simulink model "Air"  (R2026a)
settings: configuration reference "standardSILConfiguraitonParams" (kept outside this file)
undefined symbols (not defined in the file): F, gustDuration_sec, gustEnabled, gustStartTime_sec, Light, MIL, turbulenceEnabled, turbulenceEndTime_sec, turbulenceMinAirspeed_mps, turbulenceStartTime_sec, WIND_SOURCE, xWindInNED_mps, yWindInNED_mps, zWindInNED_mps
libraries: aerolibwind2 x3, simulink x2, aerolibatmos2 x1
settings Model: Creator=jerem  LastModifiedBy=Edison Altamirano
settings ConfigSetRef: SourceName=standardSILConfiguraitonParams  SourceLocation=Base Workspace

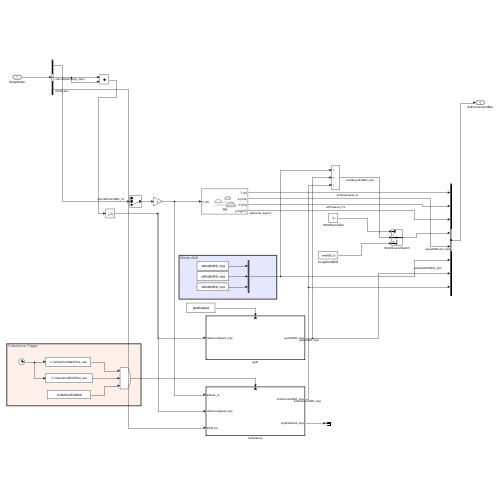
[thumbnail: Simulink's stored preview of the top-level diagram]
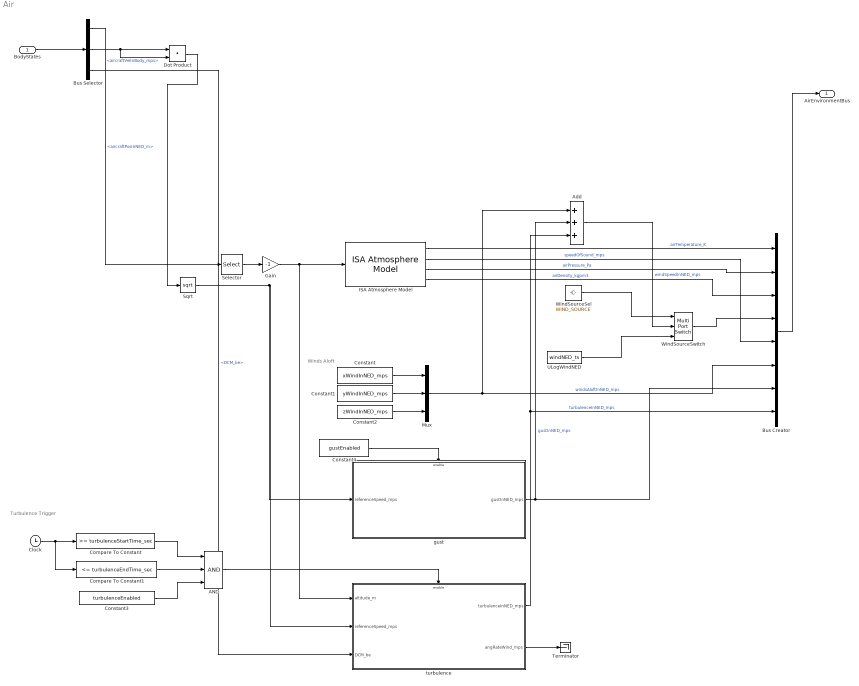
== system Air ==
  note: Turbulence Trigger
  note: Winds Aloft
  BodyStates : Inport  OutDataTypeStr=Bus: BodyStateBus
  AND : Logic  Inputs=3  IconShape=distinctive  AllPortsSameDT=off  OutDataTypeStr=boolean
  Add : Sum  Inputs=+++
  Bus Creator : BusCreator  Inputs=8  OutDataTypeStr=Bus: AirEnvironmentBus
  Bus Selector : BusSelector  OutputSignals=aircraftPosInNED_m,aircraftVelInBody_mps,DCM_be
  Clock : Clock
  Compare To Constant : simulink/Logic and Bit Operations/Compare To Constant  relop=>=  const=turbulenceStartTime_sec  OutDataTypeStr=boolean
  Compare To Constant1 : simulink/Logic and Bit Operations/Compare To Constant  relop=<=  const=turbulenceEndTime_sec  OutDataTypeStr=boolean
  Constant : Constant  Value=xWindInNED_mps
  Constant1 : Constant  Value=yWindInNED_mps
  Constant2 : Constant  Value=zWindInNED_mps
  Constant3 : Constant  Value=turbulenceEnabled
  Constant4 : Constant  Value=gustEnabled
  Dot Product : DotProduct  OutDataTypeStr=Inherit: Inherit via internal rule
  Gain : Gain  Gain=-1
  ISA Atmosphere Model : aerolibatmos2/ISA Atmosphere Model  useExtended=off  action=Warning  custom=off  viscosityOut=off  g=9.80665  gamma=1.4  R=287.0531  L=0.0065  h_trop=11000  h_strat=20000  rho0=1.225  P0=101325  T0=288.15  h0=0  S=110.4  Tref=273.15  muref=1.716e-5
  Mux : Mux  Inputs=3
  Selector : Selector  InputPortWidth=3  IndexOptions=Index vector (dialog)  Indices=3  OutputSizes=1
  Sqrt : Sqrt
  Terminator : Terminator
  ULogWindNED : FromWorkspace  VariableName=windNED_ts  OutputAfterFinalValue=Holding final value
  WindSourceSel : Constant  Value=WIND_SOURCE
  WindSourceSwitch : MultiPortSwitch  Inputs=2  SaturateOnIntegerOverflow=off  InputSameDT=off
  gust : Subsystem
  turbulence : Subsystem
  AirEnvironmentBus : Outport  OutDataTypeStr=Bus: AirEnvironmentBus
  wires:
  Constant1/1 -> Mux/2
  Constant/1 -> Mux/1
  Constant2/1 -> Mux/3
  Bus Creator/1 -> AirEnvironmentBus/1
  Selector/1 -> Gain/1
  ISA Atmosphere Model/3 -> Bus Creator/2  "airPressure_Pa"
  Bus Selector/1 -> Selector/1  "<aircraftPosInNED_m>"
  Gain/1 -> turbulence/1(altitude_m), ISA Atmosphere Model/1
  ISA Atmosphere Model/2 -> Bus Creator/5  "speedOfSound_mps"
  ISA Atmosphere Model/1 -> Bus Creator/1  "airTemperature_K"
  BodyStates/1 -> Bus Selector/1
  Mux/1 -> Bus Creator/6, Add/1  "windsAloftInNED_mps"
  ISA Atmosphere Model/4 -> Bus Creator/3  "airDensity_kgpm3"
  gust/1(gustInNED_mps) -> Bus Creator/7, Add/2  "gustInNED_mps"
  Add/1 -> WindSourceSwitch/2  "windSpeedInNED_mps"
  Bus Selector/2 -> Dot Product/2, Dot Product/1  "<aircraftVelInBody_mps>"
  Dot Product/1 -> Sqrt/1
  Bus Selector/3 -> turbulence/3(DCM_be)  "<DCM_be>"
  turbulence/1(turbulenceInNED_mps) -> Bus Creator/8, Add/3  "turbulenceInNED_mps"
  turbulence/2(angRateWind_mps) -> Terminator/1
  Sqrt/1 -> gust/1(referenceSpeed_mps), turbulence/2(referenceSpeed_mps)
  Clock/1 -> Compare To Constant1/1, Compare To Constant/1
  Compare To Constant/1 -> AND/1
  Compare To Constant1/1 -> AND/2
  AND/1 -> turbulence/Enable
  Constant3/1 -> AND/3
  Constant4/1 -> gust/Enable
  WindSourceSel/1 -> WindSourceSwitch/1
  ULogWindNED/1 -> WindSourceSwitch/3
  WindSourceSwitch/1 -> Bus Creator/4

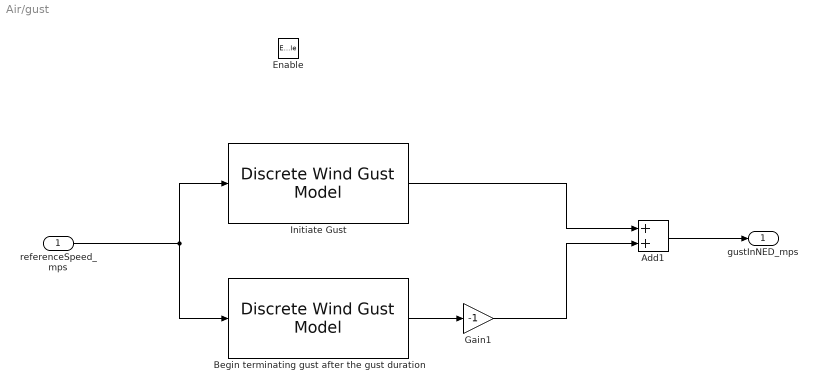
== system Air/gust ==
  referenceSpeed_mps : Inport
  Enable : EnablePort
  Add1 : Sum
  Begin terminating gust after the gust duration : aerolibwind2/Discrete Wind Gust Model  units=Metric (MKS)  Gx=on  Gy=on  Gz=on  t_0=gustStartTime_sec + gustDuration_sec  d_m=gustLength_m  v_m=gustAmplitude_mps
  Gain1 : Gain  Gain=-1
  Initiate Gust : aerolibwind2/Discrete Wind Gust Model  units=Metric (MKS)  Gx=on  Gy=on  Gz=on  t_0=gustStartTime_sec  d_m=gustLength_m  v_m=gustAmplitude_mps
  gustInNED_mps : Outport
  wires:
  referenceSpeed_mps/1 -> Begin terminating gust after the gust duration/1, Initiate Gust/1
  Gain1/1 -> Add1/2
  Begin terminating gust after the gust duration/1 -> Gain1/1
  Initiate Gust/1 -> Add1/1
  Add1/1 -> gustInNED_mps/1

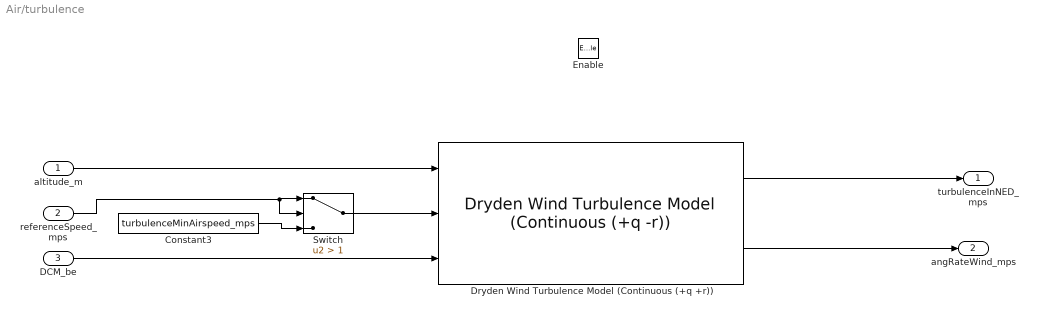
== system Air/turbulence ==
  altitude_m : Inport
  referenceSpeed_mps : Inport  Port=2
  DCM_be : Inport  Port=3
  Enable : EnablePort
  Constant3 : Constant  Value=turbulenceMinAirspeed_mps
  Dryden Wind Turbulence Model (Continuous (+q +r)) : aerolibwind2/Dryden Wind Turbulence Model  (Continuous (+q -r))  units=Metric (MKS)  spec=MIL-F-8785C  model=Continuous Dryden (+q +r)  W20=15  Wdeg=0  TurbProb=10^-2 - Light  L_high=533.4  Wingspan=turbulenceWingspan_m  ts=0.1  Seed=[23341 23342 23343 23344]  T_on=on
      settings: LibrarySourceBlock=|
      | aerolibwind2/Dryden Wind Turbulence Model
      | (Continuous (+q +r))
  Switch : Switch  Criteria=u2 > Threshold  Threshold=1  SaturateOnIntegerOverflow=off  InputSameDT=off
  turbulenceInNED_mps : Outport
  angRateWind_mps : Outport  Port=2
  wires:
  DCM_be/1 -> Dryden Wind Turbulence Model (Continuous (+q +r))/3
  Dryden Wind Turbulence Model (Continuous (+q +r))/2 -> angRateWind_mps/1
  altitude_m/1 -> Dryden Wind Turbulence Model (Continuous (+q +r))/1
  Switch/1 -> Dryden Wind Turbulence Model (Continuous (+q +r))/2
  Constant3/1 -> Switch/3
  Dryden Wind Turbulence Model (Continuous (+q +r))/1 -> turbulenceInNED_mps/1
  referenceSpeed_mps/1 -> Switch/1, Switch/2
